simulink model "zad1_sim"  (R2022b)
settings: Solver=VariableStepAuto  StartTime=0.0  StopTime=1  RelTol=1e-3
settings Model: Creator=Mat  LastModifiedBy=Mat

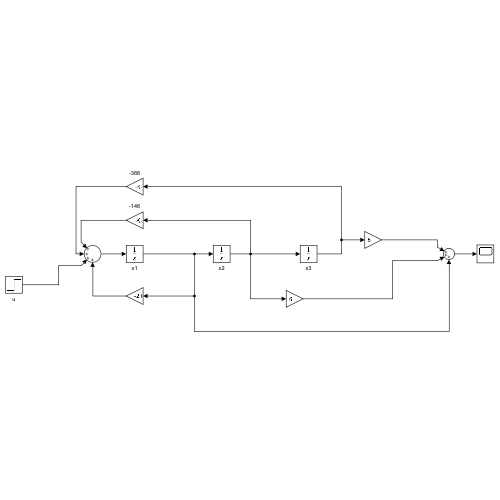
[thumbnail: Simulink's stored preview of the top-level diagram]
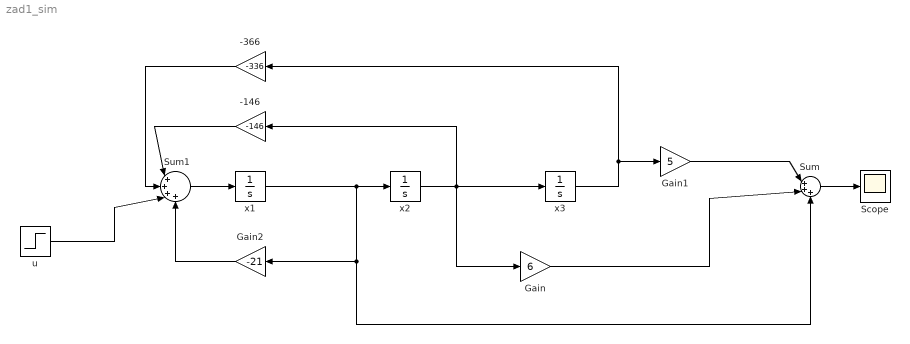
== system zad1_sim ==
  -146 : Gain  Gain=-146
  -366 : Gain  Gain=-336
  Gain : Gain  Gain=6
  Gain1 : Gain  Gain=5
  Gain2 : Gain  Gain=-21
  Scope : Scope
  Sum : Sum  Inputs=|+++
  Sum1 : Sum  Inputs=|++++
  u : Step  SampleTime=0
  x1 : Integrator  InitialCondition=-1
  x2 : Integrator  InitialCondition=-2
  x3 : Integrator  InitialCondition=-3
  wires:
  x2/1 -> -146/1, x3/1, Gain/1
  Sum/1 -> Scope/1
  x3/1 -> Gain1/1, -366/1
  Sum1/1 -> x1/1
  Gain1/1 -> Sum/1
  Gain/1 -> Sum/2
  x1/1 -> Gain2/1, Sum/3, x2/1
  Gain2/1 -> Sum1/4
  -146/1 -> Sum1/1
  -366/1 -> Sum1/2
  u/1 -> Sum1/3
